simulink model "untitled"  (R2018a)
settings: Solver=VariableStepAuto  StartTime=0.0  StopTime=10.0  RelTol=1e-3
settings Model: Creator=This PC  LastModifiedBy=This PC

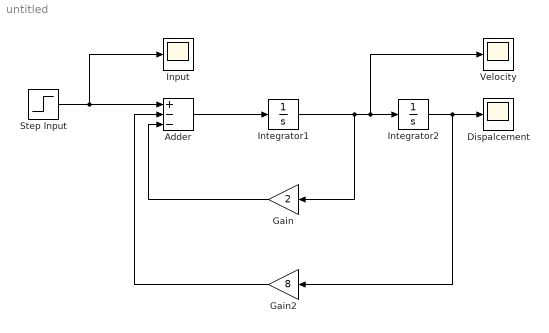
== system untitled ==
  Adder : Sum  Inputs=+--
  Dispalcement : Scope
  Gain : Gain  Gain=2
  Gain2 : Gain  Gain=8
  Input : Scope
  "Integrator1 " : Integrator  ContinuousStateAttributes=Integrator
  "Integrator2 " : Integrator
  Step Input : Step  SampleTime=0
  Velocity : Scope
  wires:
  Step Input/1 -> Input/1, Adder/1
  Adder/1 -> "Integrator1 "/1
  "Integrator1 "/1 -> Gain/1, Velocity/1, "Integrator2 "/1
  Gain/1 -> Adder/3
  Gain2/1 -> Adder/2
  "Integrator2 "/1 -> Gain2/1, Dispalcement/1
